simulink model "Accel_model"  (R2016a)
settings: Solver=VariableStepAuto  StartTime=0.0  StopTime=5  RelTol=1e-3
values from neighbouring files (symbols this model uses):
  b = 0.5    [Initialisation_variables_workspace.m]    (also in TDNaccel.m = 0.0377358490566)
  c_roul = m*g*b    (= 105.503773585)    [TDNaccel.m]
  D_roue = 0.53    [Initialisation_variables_workspace.m]    (also in TDNaccel.m)
  g = 9.81    [Initialisation_variables_workspace.m]    (also in TDNaccel.m)
  h = (mpilote*h_p + mveh*h_v)/m    (= 0.3)    [Initialisation_variables_workspace.m]
  J_eq = J_trans + 4*J_rot    (= 20.458125)    [Initialisation_variables_workspace.m]    (also in TDNaccel.m = 20.014125)
  m = mtot    (= 285)    [Initialisation_variables_workspace.m]    (also in TDNaccel.m)
  v = 1.2    [Initialisation_variables_workspace.m]    (also in TDNaccel.m = 0.133180615878)
undefined symbols (not defined in the file or in its folder): c_roue, rap1, rap2, rap3, rap4, rap5, rap6
settings Model: Creator=Aurélien  LastModifiedBy=Brice

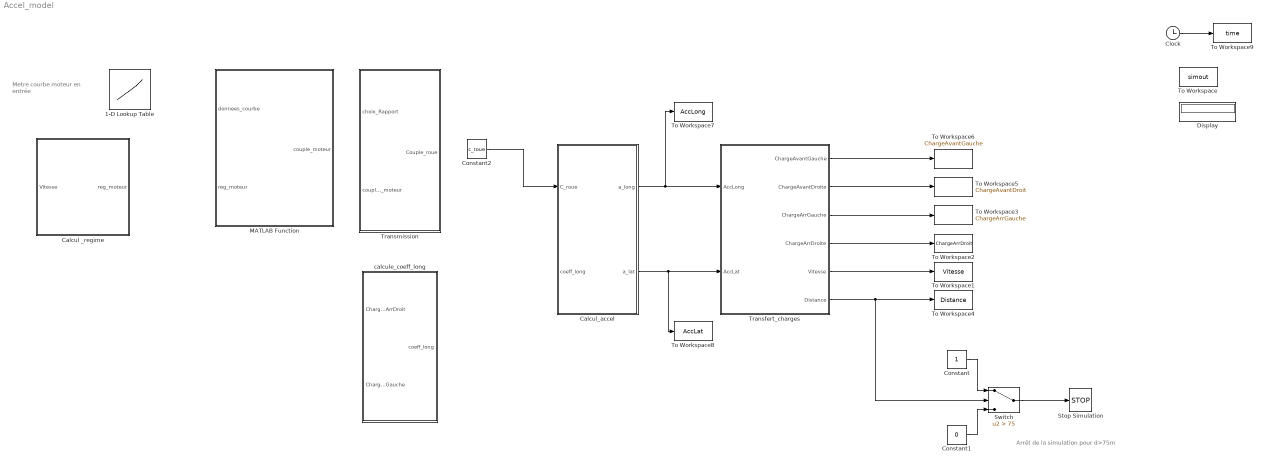
== system Accel_model ==
  note: Metre courbe moteur
      | en entrée
  note: Arrêt de la simulation pour d>75m
  1-D Lookup Table : Lookup_n-D  NumberOfTableDimensions=1  BreakpointsForDimension1=[-5:5]  Table=tanh([-5:5])  InternalRulePriority=Speed  RndMeth=Simplest  InputSameDT=on
  Calcul _regime : MATLAB Function  TreatAsAtomicUnit=on
  Calcul_accel : Subsystem
  Clock : Clock
  Constant : Constant
  Constant1 : Constant  Value=0
  Constant2 : Constant  Value=c_roue
  Display : Display
  MATLAB Function : MATLAB Function  TreatAsAtomicUnit=on
  Stop Simulation : Stop
  Switch : Switch  Criteria=u2 > Threshold  Threshold=75
  To Workspace : ToWorkspace  VariableName=simout  SaveFormat=Timeseries  SampleTime=-1
  To Workspace1 : ToWorkspace  VariableName=Vitesse  SaveFormat=Timeseries  SampleTime=-1
  To Workspace2 : ToWorkspace  VariableName=ChargeArrDroit  SaveFormat=Timeseries  SampleTime=-1
  To Workspace3 : ToWorkspace  VariableName=ChargeArrGauche  SaveFormat=Timeseries  SampleTime=-1
  To Workspace4 : ToWorkspace  VariableName=Distance  SaveFormat=Timeseries  SampleTime=-1
  To Workspace5 : ToWorkspace  VariableName=ChargeAvantDroit  SaveFormat=Timeseries  SampleTime=-1
  To Workspace6 : ToWorkspace  VariableName=ChargeAvantGauche  SaveFormat=Timeseries  SampleTime=-1
  To Workspace7 : ToWorkspace  VariableName=AccLong  SaveFormat=Timeseries  SampleTime=-1
  To Workspace8 : ToWorkspace  VariableName=AccLat  SaveFormat=Timeseries  SampleTime=-1
  To Workspace9 : ToWorkspace  VariableName=time  SampleTime=-1
  Transfert_charges : Subsystem
  Transmission : Subsystem
  calcule_coeff_long : MATLAB Function  TreatAsAtomicUnit=on
  wires:
  Transfert_charges/6(Distance) -> Switch/2, To Workspace4/1
  Switch/1 -> Stop Simulation/1
  Constant1/1 -> Switch/3
  Constant/1 -> Switch/1
  Transfert_charges/5(Vitesse) -> To Workspace1/1
  Transfert_charges/4(ChargeArrDroite) -> To Workspace2/1
  Transfert_charges/3(ChargeArrGauche) -> To Workspace3/1
  Transfert_charges/2(ChargeAvantDroite) -> To Workspace5/1
  Transfert_charges/1(ChargeAvantGauche) -> To Workspace6/1
  Calcul_accel/1(a_long) -> To Workspace7/1, Transfert_charges/1(AccLong)
  Calcul_accel/2(a_lat) -> To Workspace8/1, Transfert_charges/2(AccLat)
  Constant2/1 -> Calcul_accel/1(C_roue)
  Clock/1 -> To Workspace9/1

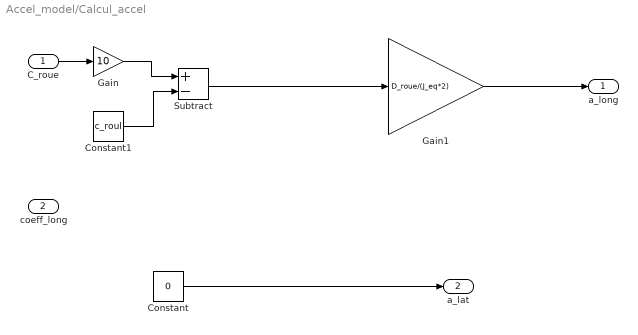
== system Accel_model/Calcul_accel ==
  C_roue : Inport
  coeff_long : Inport  Port=2
  Constant : Constant  Value=0
  Constant1 : Constant  Value=c_roul
  Gain : Gain  Gain=10
  Gain1 : Gain  Gain=D_roue/(J_eq*2)
  Subtract : Sum  Inputs=+-
  a_long : Outport
  a_lat : Outport  Port=2
  wires:
  Constant/1 -> a_lat/1
  C_roue/1 -> Gain/1
  Gain/1 -> Subtract/1
  Constant1/1 -> Subtract/2
  Gain1/1 -> a_long/1
  Subtract/1 -> Gain1/1

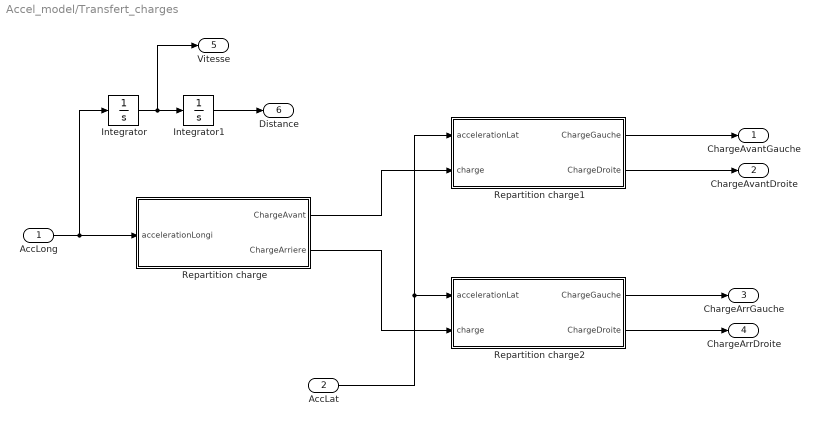
== system Accel_model/Transfert_charges ==
  AccLong : Inport
  AccLat : Inport  Port=2
  Integrator : Integrator
  Integrator1 : Integrator
  Repartition charge : Subsystem
  Repartition charge1 : Subsystem
  Repartition charge2 : Subsystem
  ChargeAvantGauche : Outport
  ChargeAvantDroite : Outport  Port=2
  ChargeArrGauche : Outport  Port=3
  ChargeArrDroite : Outport  Port=4
  Vitesse : Outport  Port=5
  Distance : Outport  Port=6
  wires:
  Repartition charge/1(ChargeAvant) -> Repartition charge1/2("charge ")
  Repartition charge/2(ChargeArriere) -> Repartition charge2/2("charge ")
  AccLong/1 -> Integrator/1, Repartition charge/1(accelerationLongi)
  AccLat/1 -> Repartition charge1/1(accelerationLat), Repartition charge2/1(accelerationLat)
  Integrator/1 -> Vitesse/1, Integrator1/1
  Integrator1/1 -> Distance/1
  Repartition charge1/2(ChargeDroite) -> ChargeAvantDroite/1
  Repartition charge1/1(ChargeGauche) -> ChargeAvantGauche/1
  Repartition charge2/1(ChargeGauche) -> ChargeArrGauche/1
  Repartition charge2/2(ChargeDroite) -> ChargeArrDroite/1

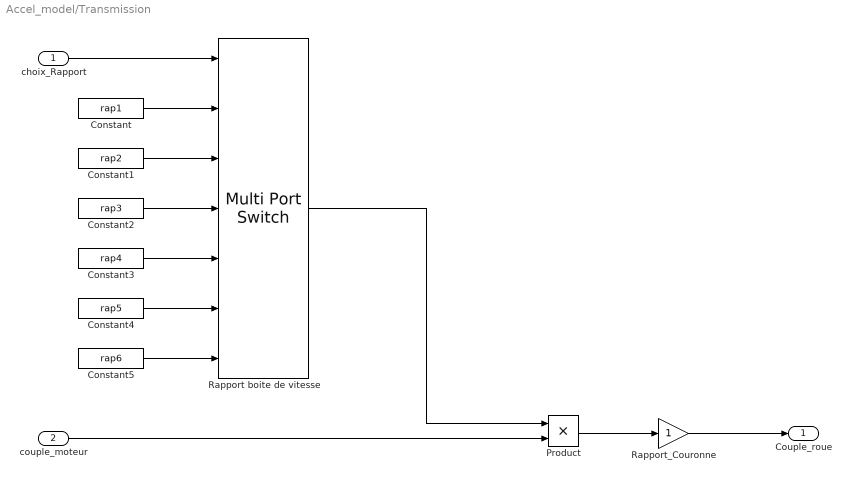
== system Accel_model/Transmission ==
  choix_Rapport : Inport
  couple_moteur : Inport  Port=2
  Constant : Constant  Value=rap1
  Constant1 : Constant  Value=rap2
  Constant2 : Constant  Value=rap3
  Constant3 : Constant  Value=rap4
  Constant4 : Constant  Value=rap5
  Constant5 : Constant  Value=rap6
  Product : Product
  Rapport boite de vitesse : MultiPortSwitch  Inputs=6
  Rapport_Couronne : Gain
  Couple_roue : Outport
  wires:
  Constant/1 -> Rapport boite de vitesse/2
  Constant1/1 -> Rapport boite de vitesse/3
  Constant2/1 -> Rapport boite de vitesse/4
  Constant3/1 -> Rapport boite de vitesse/5
  Constant4/1 -> Rapport boite de vitesse/6
  choix_Rapport/1 -> Rapport boite de vitesse/1
  Rapport boite de vitesse/1 -> Product/1
  couple_moteur/1 -> Product/2
  Rapport_Couronne/1 -> Couple_roue/1
  Product/1 -> Rapport_Couronne/1
  Constant5/1 -> Rapport boite de vitesse/7

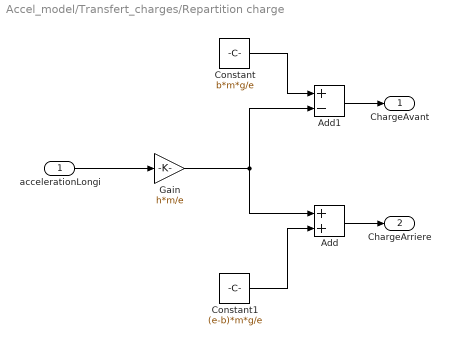
== system Accel_model/Transfert_charges/Repartition charge ==
  accelerationLongi : Inport
  Add : Sum
  Add1 : Sum  Inputs=+-
  Constant : Constant  Value=b*m*g/e
  Constant1 : Constant  Value=(e-b)*m*g/e
  Gain : Gain  Gain=h*m/e
  ChargeAvant : Outport
  ChargeArriere : Outport  Port=2
  wires:
  accelerationLongi/1 -> Gain/1
  Gain/1 -> Add/1, Add1/2
  Constant/1 -> Add1/1
  Constant1/1 -> Add/2
  Add1/1 -> ChargeAvant/1
  Add/1 -> ChargeArriere/1

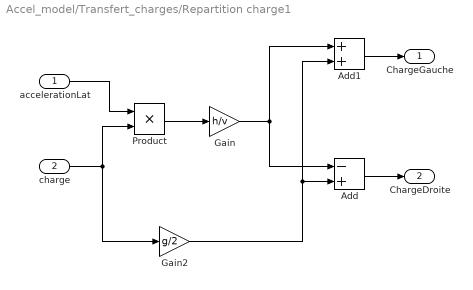
== system Accel_model/Transfert_charges/Repartition charge1 ==
  accelerationLat : Inport
  "charge " : Inport  Port=2
  Add : Sum  Inputs=-+
  Add1 : Sum
  Gain : Gain  Gain=h/v
  Gain2 : Gain  Gain=g/2
  Product : Product
  ChargeGauche : Outport
  ChargeDroite : Outport  Port=2
  wires:
  Gain/1 -> Add1/1, Add/1
  Add1/1 -> ChargeGauche/1
  Add/1 -> ChargeDroite/1
  accelerationLat/1 -> Product/1
  "charge "/1 -> Product/2, Gain2/1
  Product/1 -> Gain/1
  Gain2/1 -> Add1/2, Add/2

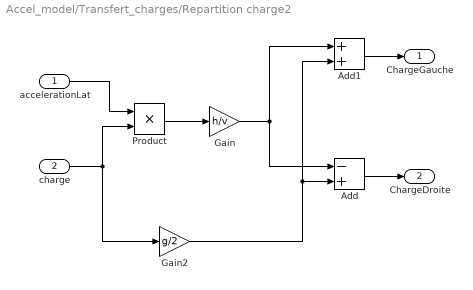
== system Accel_model/Transfert_charges/Repartition charge2 ==
  accelerationLat : Inport
  "charge " : Inport  Port=2
  Add : Sum  Inputs=-+
  Add1 : Sum
  Gain : Gain  Gain=h/v
  Gain2 : Gain  Gain=g/2
  Product : Product
  ChargeGauche : Outport
  ChargeDroite : Outport  Port=2
  wires:
  Gain/1 -> Add1/1, Add/1
  Add1/1 -> ChargeGauche/1
  Add/1 -> ChargeDroite/1
  accelerationLat/1 -> Product/1
  "charge "/1 -> Product/2, Gain2/1
  Product/1 -> Gain/1
  Gain2/1 -> Add1/2, Add/2

== matlab function Accel_model/Calcul _regime ==
  data: Vitesse input; reg_moteur output
function reg_moteur = fcn(Vitesse)
%#codegen

y = u;

== matlab function Accel_model/calcule_coeff_long ==
  data: ChargeArrDroit input; coeff_long output; ChargeArrGauche input
function coeff_long = fcn(ChargeArrDroit,ChargeArrGauche)
%#codegen

y = u;

== matlab function Accel_model/MATLAB Function ==
  data: donnees_courbe input; couple_moteur output; reg_moteur input
function couple_moteur = fcn(donnees_courbe,reg_moteur)
%#codegen

y = u;
